simulink model "sldemo_absbrake"  (R2023b)
settings: Solver=FixedStepAuto  StartTime=0.0  StopTime=25  FixedStep=0.01  MaxStep=.01  RelTol=1e-3  AbsTol=1e-6
PreLoadFcn:
  | % Load initialization data
  | 
  | sldemo_absdata;
StopFcn:
  |  if exist ('sldemo_absbrake_output')
  |  sldemo_absbrakeplots;
  |  end
undefined symbols (not defined in the file): ctrl, DiscIntNeverNeededParam, g, m, mu, Rr, slip, v0
CloseFcn:
  | % Close the plots that are still open
  | h = findobj(0, 'Name', 'ABS Speeds');
  | if ~isempty(h),
  |   close(h);
  | end;
  | 
  | h = findobj(0, 'Name', 'ABS Slip');
  | if ~isempty(h),
  |   close(h);
  | end;
  | 
  | % Clear initial conditions data to avoid cluttering the workspace
  | 
  | clear g v0 Rr Kf m PBmax TB I slip mu ctrl h;
Description:
  | Modeling an Anti-Lock Braking System (ABS)
  | 
  | *Summary*
  | 
  | This example describes a simple model for an Anti-Lock Braking System
  | (ABS). The model simulates the dynamic behavior of a vehicle
  | under hard braking conditions. The model represents a single wheel, which
  | may be replicated a number of times to create a model for a multi-wheel
  | vehicle.
  | 
  | This model uses the signal logging feature in Simulink(R). You log signals to the
  | MATLAB(R) workspace where you can analyze and view them. You can view
  | the code in sldemo_absbrakeplots.m to see how this is done.
  | 
  | In this model, the wheel speed is calculated in a separate component
  | named sldemo_wheelspeed_absbrake.
  | This component is then referenced using a Model block.  Note that both the
  | top model and the referenced model use a variable step solver, so Simulink
  | will track zero-crossings in the referenced model.
settings Model: FPTRunName=Active  ModifiedByFormat=The MathWorks, Inc.  Creator=The MathWorks, Inc.  LastModifiedBy=The MathWorks, Inc.
settings SolverCC: AutoScaleAbsTol=off  AlgebraicLoopSolver=TrustRegion  MaxZcPerStep=1
settings DataIOCC: SaveFormat=Array  SaveOutput=off  SaveTime=off  ReturnWorkspaceOutputs=off  TimeSaveName=time  SignalLoggingName=sldemo_absbrake_output
settings OptimizationCC: DefaultParameterBehavior=Inlined  UseDivisionForNetSlopeComputation=on  InlineInvariantSignals=on  EnhancedBackFolding=on  PassReuseOutputArgsAs=Individual arguments  ExpressionDepthLimit=2147483647  StateBitsets=on  DataBitsets=on  ZeroExternalMemoryAtStartup=off  ZeroInternalMemoryAtStartup=off  EfficientFloat2IntCast=on  LifeSpan=inf  BufferReusableBoundary=off  OptimizeBlockOrder=speed  DifferentSizesBufferReuse=on  EfficientTunableParamExpr=on
settings DebuggingCC: SignalInfNanChecking=warning  SaveWithParameterizedLinksMsg=none  SigSpecEnsureSampleTimeMsg=none  IntegerOverflowMsg=error  ParameterTunabilityLossMsg=error  UnconnectedInputMsg=warning  UnconnectedOutputMsg=warning  UnconnectedLineMsg=warning  UniqueDataStoreMsg=error  BusObjectLabelMismatch=none  AssertControl=DisableAll  AllowSymbolicDim=off  StateNameClashWarn=warning  SubsystemReferenceDiagnosticForUnitTest=warning  SFUnexpectedBacktrackingDiag=warning  SFNoUnconditionalDefaultTransitionDiag=warning  SFUndirectedBroadcastEventsDiag=error  SFExecutionAtInitializationDiag=none  IntegerSaturationMsg=none  ArithmeticOperatorsInVariantConditions=warning
settings HardwareCC: ProdBitPerPointer=32  ProdBitPerSizeT=32  ProdBitPerPtrDiffT=32  ProdLargestAtomicFloat=None  ProdEndianess=Unspecified  ProdWordSize=32  ProdHWDeviceType=32-bit Generic  TargetBitPerPointer=64  TargetBitPerSizeT=64  TargetBitPerPtrDiffT=64  TargetLongLongMode=on  TargetIntDivRoundTo=Zero  TargetEndianess=LittleEndian  TargetWordSize=64  TargetHWDeviceType=MATLAB Host
settings ModelReferenceCC: UpdateModelReferenceTargets=IfOutOfDate  EnableRefExpFcnMdlSchedulingChecks=on  PropagateSignalLabelsOutOfModel=off
settings SFSimCC: SimUseLocalCustomCode=off  CompileTimeRecursionLimit=0  EnableRuntimeRecursion=off  MATLABDynamicMemAlloc=off  CustomCodeUndefinedFunction=UseInterfaceOnly
settings RTWCC: Description=Embedded Coder  SystemTargetFile=ert.tlc  TemplateMakefile=ert_default_tmf  RTWUseLocalCustomCode=off  DLArmComputeVersion=19.05
settings CodeAppCC: ForceParamTrailComments=on  IgnoreCustomStorageClasses=off  IgnoreTestpoints=on  OperatorAnnotations=on  SimulinkDataObjDesc=on  SFDataObjDesc=on  MATLABFcnDesc=on  InsertBlockDesc=on
settings ERTTargetCC: UtilityFuncGeneration=Shared location  GenerateSampleERTMain=on  SupportAbsoluteTime=off  ParenthesesLevel=Standards  CastingMode=Standards  GenerateSharedConstants=off  InlinedParameterPlacement=NonHierarchical  ERTCustomFileTemplate=example_file_process.tlc  SuppressUnreachableDefaultCases=off  EnableSignedLeftShifts=off  EnableSignedRightShifts=off
settings ConfigComp: CovMetricSettings=dw  CovSaveCumulativeToWorkspaceVar=on  CovSaveSingleToWorkspaceVar=on  CovExternalEMLEnable=off  CovSFcnEnable=off

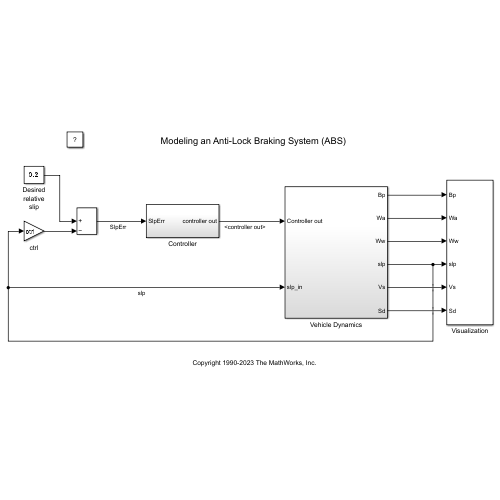
[thumbnail: Simulink's stored preview of the top-level diagram]
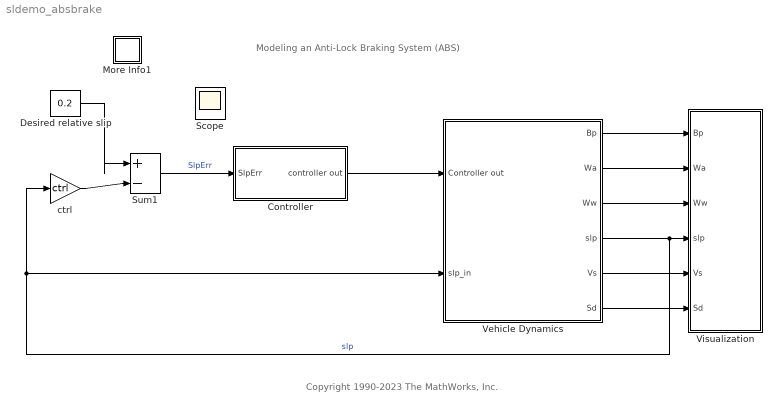
== system sldemo_absbrake ==
  note: Modeling an Anti-Lock Braking System (ABS)
  note: Copyright 1990-2023 The MathWorks, Inc.
  Controller : Subsystem
  Desired relative slip : Constant  Value=0.2
  More Info1 : Subsystem
      settings: OpenFcn=showExample('simulink_automotive/ModelingAnAntiLockBrakingSystemExample')
      mask Display: disp('?')
  Sum1 : Sum  Inputs=|+-  InputSameDT=on  SaturateOnIntegerOverflow=on  OutDataTypeStr=Inherit: Same as first input
  Vehicle Dynamics : Subsystem
  Visualization : Subsystem
  ctrl : Gain  Gain=ctrl
  Scope : Scope
  wires:
  Sum1/1 -> Controller/1(SlpErr)  "SlpErr"
  Desired relative slip/1 -> Sum1/1
  ctrl/1 -> Sum1/2
  Vehicle Dynamics/4(slp) -> Visualization/4(slp), ctrl/1, Vehicle Dynamics/2(slp_in)  "slp"
  Controller/1(controller out) -> Vehicle Dynamics/1(Controller out)
  Vehicle Dynamics/1(Bp) -> Visualization/1(Bp)
  Vehicle Dynamics/2(Wa) -> Visualization/2(Wa)
  Vehicle Dynamics/3(Ww) -> Visualization/3(Ww)
  Vehicle Dynamics/5(Vs) -> Visualization/5(Vs)
  Vehicle Dynamics/6(Sd) -> Visualization/6(Sd)

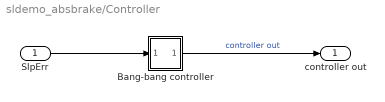
== system sldemo_absbrake/Controller ==
  SlpErr : Inport
  Bang-bang controller : Subsystem  mask(Sign){}
      mask help: y = sign(x)
      mask Help: Sign Function:\n\t\t\ty = 1 if x > 0\n\t\t\ty = 0 if x = 0\n\t\t\ty = -1 if x < 0
      mask Display: plot(-50,-50,50,50,[-50,50],[0,0],[0,0],[-50,50],[-40,0],[-30,-30],[0,40],[30,30])
  controller out : Outport
  wires:
  Bang-bang controller/1(out_1) -> controller out/1  "controller out"
  SlpErr/1 -> Bang-bang controller/1(in_1)

== system sldemo_absbrake/More Info1 ==

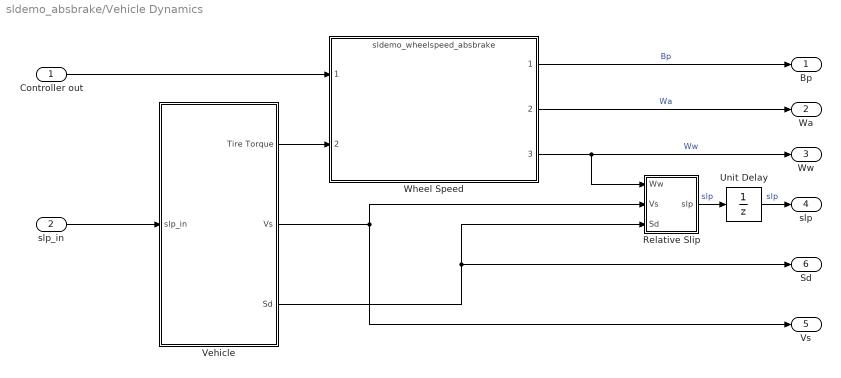
== system sldemo_absbrake/Vehicle Dynamics ==
  Controller out : Inport
  slp_in : Inport  Port=2
  Relative Slip : Subsystem
  Unit Delay : UnitDelay  SampleTime=-1  HasFrameUpgradeWarning=on
  "Vehicle  " : Subsystem
  Wheel Speed : ModelReference  ModelNameDialog=sldemo_wheelspeed_absbrake.slx  SimulationMode=Normal  ModelReferenceVersion=7.40
  Bp : Outport
  Wa : Outport  Port=2
  Ww : Outport  Port=3
  slp : Outport  Port=4
  Vs : Outport  Port=5
  Sd : Outport  Port=6
  wires:
  Wheel Speed/3 -> Relative Slip/1(Ww), Ww/1  "Ww"
  "Vehicle  "/2(Vs) -> Vs/1, Relative Slip/2(Vs)
  "Vehicle  "/1(Tire Torque) -> Wheel Speed/2
  "Vehicle  "/3(Sd) -> Relative Slip/3(Sd), Sd/1
  Relative Slip/1(slp) -> Unit Delay/1  "slp"
  Controller out/1 -> Wheel Speed/1
  Wheel Speed/1 -> Bp/1  "Bp"
  slp_in/1 -> "Vehicle  "/1(slp_in)
  Wheel Speed/2 -> Wa/1  "Wa"
  Unit Delay/1 -> slp/1  "slp"

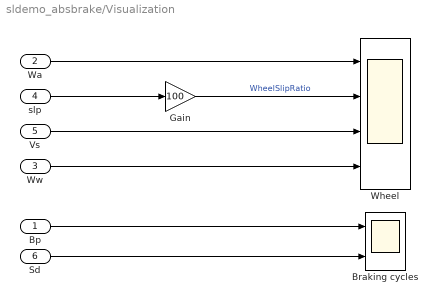
== system sldemo_absbrake/Visualization ==
  Bp : Inport
  Wa : Inport  Port=2
  Ww : Inport  Port=3
  slp : Inport  Port=4
  Vs : Inport  Port=5
  Sd : Inport  Port=6
  Braking cycles : Scope  NumInputPorts=2
  Gain : Gain  Gain=100
  Wheel : Scope  NumInputPorts=4
  wires:
  Bp/1 -> Braking cycles/1
  Wa/1 -> Wheel/1
  Ww/1 -> Wheel/4
  Sd/1 -> Braking cycles/2
  Vs/1 -> Wheel/3
  Gain/1 -> Wheel/2  "WheelSlipRatio"
  slp/1 -> Gain/1

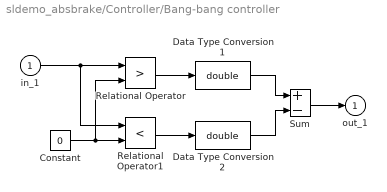
== system sldemo_absbrake/Controller/Bang-bang controller ==
  in_1 : Inport
  Constant : Constant  Value=0
  Data Type Conversion1 : DataTypeConversion  OutDataTypeStr=double
  Data Type Conversion2 : DataTypeConversion  OutDataTypeStr=double
  Relational Operator : RelationalOperator  Operator=>  OutDataTypeStr=boolean
  Relational Operator1 : RelationalOperator  Operator=<  OutDataTypeStr=boolean
  Sum : Sum  Inputs=+-  InputSameDT=on  SaturateOnIntegerOverflow=on  OutDataTypeStr=Inherit: Same as first input
  out_1 : Outport  InitialOutput=0  VectorParamsAs1DForOutWhenUnconnected=off
  wires:
  Data Type Conversion2/1 -> Sum/2
  Data Type Conversion1/1 -> Sum/1
  Sum/1 -> out_1/1
  Relational Operator/1 -> Data Type Conversion1/1
  Relational Operator1/1 -> Data Type Conversion2/1
  Constant/1 -> Relational Operator/2, Relational Operator1/2
  in_1/1 -> Relational Operator1/1, Relational Operator/1

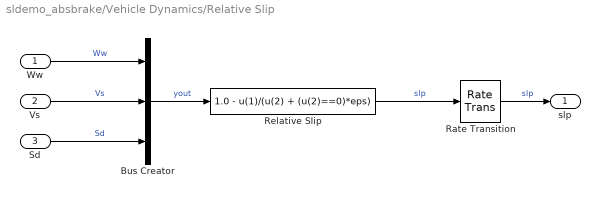
== system sldemo_absbrake/Vehicle Dynamics/Relative Slip ==
  Ww : Inport
  Vs : Inport  Port=2
  Sd : Inport  Port=3
  Bus Creator : BusCreator  Inputs=3
  Rate Transition : RateTransition  OutPortSampleTimeOpt=Inherit
  Relative Slip : Fcn  Expr=1.0 - u(1)/(u(2) + (u(2)==0)*eps)
  slp : Outport
  wires:
  Bus Creator/1 -> Relative Slip/1  "yout"
  Relative Slip/1 -> Rate Transition/1  "slp"
  Ww/1 -> Bus Creator/1  "Ww"
  Vs/1 -> Bus Creator/2  "Vs"
  Sd/1 -> Bus Creator/3  "Sd"
  Rate Transition/1 -> slp/1  "slp"

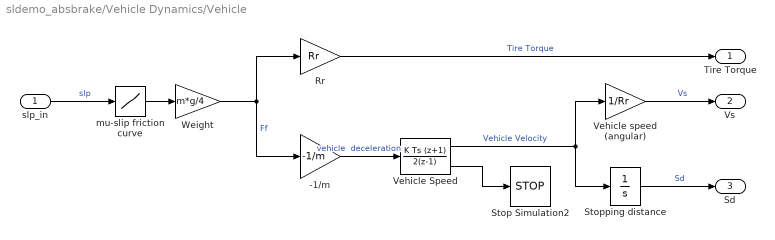
== system sldemo_absbrake/Vehicle Dynamics/Vehicle   ==
  slp_in : Inport
  -1/m : Gain  Gain=-1/m  SaturateOnIntegerOverflow=on  OutDataTypeStr=Inherit: Same as input  ParamDataTypeStr=Inherit: Same as input
  Rr : Gain  Gain=Rr  SaturateOnIntegerOverflow=on  OutDataTypeStr=Inherit: Same as input  ParamDataTypeStr=Inherit: Same as input
  Stop Simulation2 : Stop
  Stopping distance : Integrator  UpperSaturationLimit=1000  LowerSaturationLimit=0
  Vehicle Speed : DiscreteIntegrator  IntegratorMethod=Integration: Trapezoidal  InitialCondition=v0  SampleTime=-1  LimitOutput=on  UpperSaturationLimit=1000  LowerSaturationLimit=0  ShowSaturationPort=on  ICPrevOutput=DiscIntNeverNeededParam  ICPrevScaledInput=DiscIntNeverNeededParam
  Vehicle speed (angular) : Gain  Gain=1/Rr  SaturateOnIntegerOverflow=on  OutDataTypeStr=Inherit: Same as input  ParamDataTypeStr=Inherit: Same as input
  Weight : Gain  Gain=m*g/4  SaturateOnIntegerOverflow=on  OutDataTypeStr=Inherit: Same as input  ParamDataTypeStr=Inherit: Same as input
  mu-slip friction curve : Lookup_n-D  NumberOfTableDimensions=1  BreakpointsForDimension1=slip  Table=mu  SaturateOnIntegerOverflow=on
  Tire Torque : Outport  Unit=N*m
  Vs : Outport  Port=2  Unit=rad/sec
  Sd : Outport  Port=3  Unit=m
  wires:
  slp_in/1 -> mu-slip friction curve/1  "slp"
  Rr/1 -> Tire Torque/1  "Tire Torque"
  -1/m/1 -> Vehicle Speed/1  "vehicle  deceleration"
  Vehicle speed (angular)/1 -> Vs/1  "Vs"
  Stopping distance/1 -> Sd/1  "Sd"
  Weight/1 -> -1/m/1, Rr/1  "Ff"
  mu-slip friction curve/1 -> Weight/1
  Vehicle Speed/1 -> Stopping distance/1, Vehicle speed (angular)/1  "Vehicle Velocity"
  Vehicle Speed/2 -> Stop Simulation2/1
